simulink model "Traction_Test"  (R2019b)
settings: configuration reference "ConfigSet_TractionSystem_Reference" (kept outside this file)
PostLoadFcn:
  | set_up_test_model()
undefined symbols (not defined in the file): DiscIntNeverNeededParam, ElectricalSystem, Enabled, MaxVehicles, Orientation, Type, VehicleType, WheelDiameter, Z_TractionSystemPrm
libraries: TestBenchLib x27, simulink x2, VectorOperationsLib x1, MathOperationsLib x1
settings Model: EnablePacing=on  PacingRate=0.100000  OrderedModelArguments=off  Creator=lonkaran  LastModifiedBy=ext-nadpurob
settings ConfigSetRef: SourceName=ConfigSet_TractionSystem_Reference  SourceLocation=Base Workspace

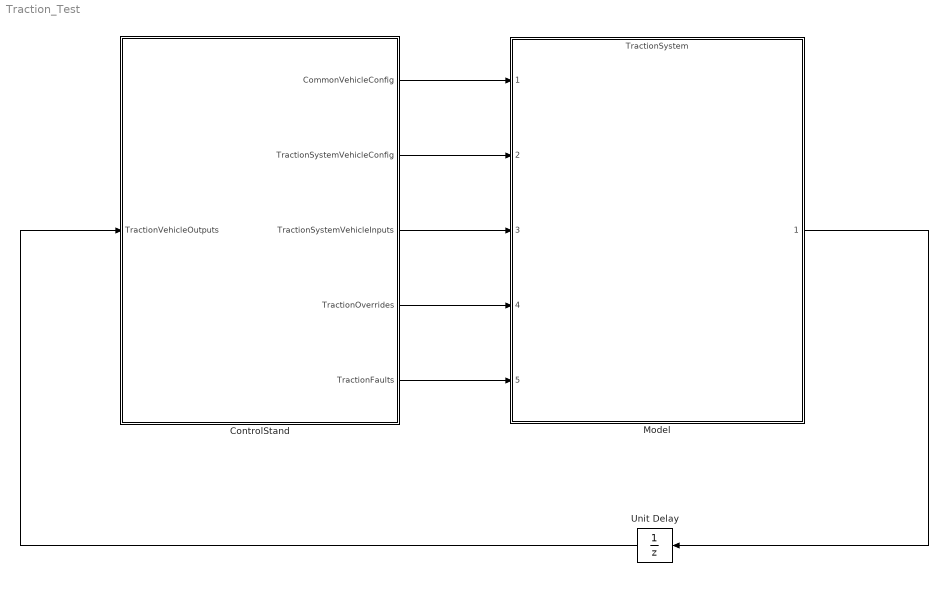
== system Traction_Test ==
  ControlStand : Subsystem
  Model : ModelReference  ModelNameDialog=TractionSystem.slx  ParameterArgumentNames=Prm_TractionSystem  ParameterArgumentValues=[Z_TractionSystemPrm]  UsingDefaultArgumentValue=0  SimulationMode=Normal  ModelReferenceVersion=1.647
  Unit Delay : UnitDelay  SampleTime=-1  HasFrameUpgradeWarning=on
  wires:
  Model/1 -> Unit Delay/1
  Unit Delay/1 -> ControlStand/1(TractionVehicleOutputs)
  ControlStand/1(CommonVehicleConfig) -> Model/1
  ControlStand/2(TractionSystemVehicleConfig) -> Model/2
  ControlStand/3(TractionSystemVehicleInputs) -> Model/3
  ControlStand/4(TractionOverrides) -> Model/4
  ControlStand/5(TractionFaults) -> Model/5

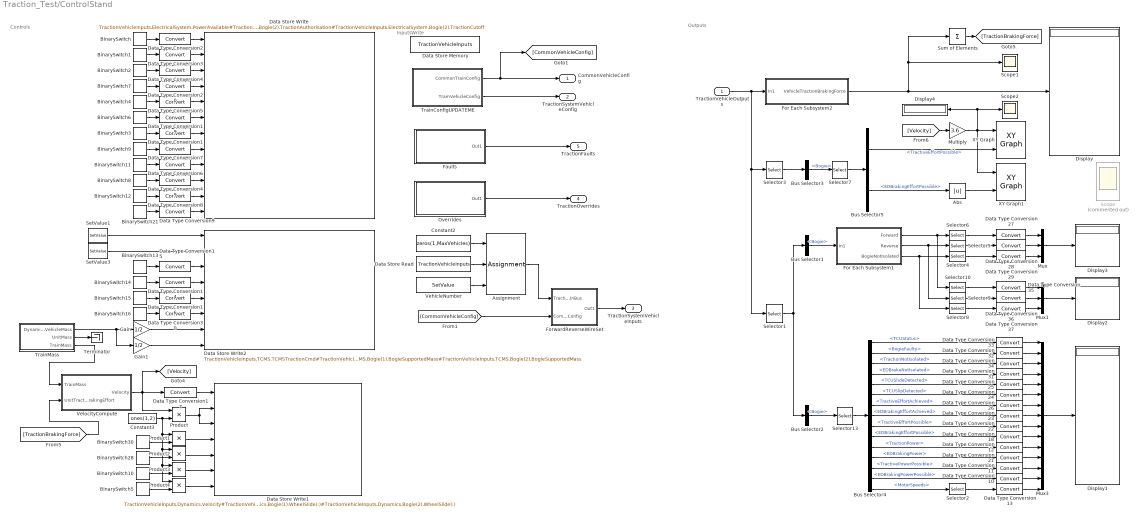
== system Traction_Test/ControlStand ==
  note: Outputs
  note: InputsWrite
  note: Controls
  TractionVehicleOutputs : Inport
  Abs : Abs
  Assignment : Assignment  DiagnosticForDimensions=Warning  IndexOptions=Index vector (port)  Indices=1  OutputSizes=1
  BinarySwitch{,1,3..4,6..9,12} (9 alike) : TestBenchLib/BinarySwitch  value=1  init_value=1  block_colour=[0 1 0]  WorkspaceVarName=0
      settings: SourceProductName=Sydac Utilities
  BinarySwitch{2,5,10..11,13..16,21,28,30} (11 alike) : TestBenchLib/BinarySwitch  value=0  init_value=0  block_colour=[0 1 0]  WorkspaceVarName=0
      settings: SourceProductName=Sydac Utilities
  Bus Selector1 : BusSelector  OutputSignals=TractionControl.ElectricalSystem.Bogie
  Bus Selector2 : BusSelector  OutputSignals=TractionControl.TCMS.Bogie
  Bus Selector3 : BusSelector  OutputSignals=TractionControl.TCMS.Bogie
  Bus Selector4 : BusSelector  OutputSignals=TCUStatus,BogieFaulty,TractionNotIsolated,EDBrakeNotIsolated,TCUSlideDetected,TCUSlipDetected,TractiveEffortAchieved,EDBrakingEffortAchieved,TractiveEffortPossible,EDBrakingEffortPossible,TractionPower,EDBrakingPower,TractivePowerPossible,EDBrakingPowerPossible,MotorSpeeds
  Bus Selector5 : BusSelector  OutputSignals=TractiveEffortPossible,EDBrakingEffortPossible
  Constant2 : Constant  Value=zeros(1,MaxVehicles)  OutDataTypeStr=Bus: BD_TractionSystem_In_Vehicle
  Constant3 : Constant  Value=ones(1,2)
  Data Store Memory : DataStoreMemory  DataStoreName=TractionVehicleInputs  ReadBeforeWriteMsg=warning  WriteAfterWriteMsg=warning  WriteAfterReadMsg=warning  ShowAdditionalParam=off  OutDataTypeStr=Bus: BD_TractionSystem_In_Vehicle
  Data Store Read : DataStoreRead  DataStoreName=TractionVehicleInputs  DataStoreElements=TractionVehicleInputs
  Data Store Write : DataStoreWrite  DataStoreName=TractionVehicleInputs  DataStoreElements=TractionVehicleInputs.ElectricalSystem.PowerAvailable#TractionVehicleInputs.ElectricalSystem.ForwardTW#TractionVehicleInputs.ElectricalSystem.ReverseTW#TractionVehicleInputs.ElectricalSystem.TractionActiveTW#TractionVehicleInputs.ElectricalSystem.NoEmergencyBrakeActiveTW#TractionVehicleInputs.ElectricalSystem.VCBState#TractionVehicleInputs.ElectricalSystem.Bogie(1).TCUPower#TractionVehicleInputs.ElectricalSystem.Bogie(1).TractionAuthorisation#TractionVehicleInputs.ElectricalSystem.Bogie(1).TractionCutoff#TractionVehicleInputs.ElectricalSystem.Bogie(2).TCUPower#TractionVehicleInputs.ElectricalSystem.Bogie(2).TractionAuthorisation#TractionVehicleInputs.ElectricalSystem.Bogie(2).TractionCutoff
  Data Store Write1 : DataStoreWrite  DataStoreName=TractionVehicleInputs  DataStoreElements=TractionVehicleInputs.Dynamics.Velocity#TractionVehicleInputs.Dynamics.Bogie(1).WheelSpeed(:)#TractionVehicleInputs.Dynamics.Bogie(2).WheelSpeed(:)#TractionVehicleInputs.Dynamics.Bogie(1).WheelSlip(:)#TractionVehicleInputs.Dynamics.Bogie(2).WheelSlip(:)#TractionVehicleInputs.Dynamics.Bogie(1).WheelSlide(:)#TractionVehicleInputs.Dynamics.Bogie(2).WheelSlide(:)
  Data Store Write2 : DataStoreWrite  DataStoreName=TractionVehicleInputs  DataStoreElements=TractionVehicleInputs.TCMS.TCMSTractionCmd#TractionVehicleInputs.TCMS.TCMSEDBrakingCmd#TractionVehicleInputs.TCMS.Bogie(1).TCMSTractionInhibit#TractionVehicleInputs.TCMS.Bogie(2).TCMSTractionInhibit#TractionVehicleInputs.TCMS.Bogie(1).TCMSDynamicBrakingInhibit#TractionVehicleInputs.TCMS.Bogie(2).TCMSDynamicBrakingInhibit#TractionVehicleInputs.TCMS.Bogie(1).BogieSupportedMass#TractionVehicleInputs.TCMS.Bogie(2).BogieSupportedMass
  Data Type Conversion{1..37,49} (38 alike) : DataTypeConversion
  Display{,1..4} (5 alike) : Display
  Faults : Subsystem
  For Each Subsystem1 : Subsystem  TreatAsAtomicUnit=on
  For Each Subsystem2 : Subsystem  TreatAsAtomicUnit=on
  ForwardReverseWireSet : Subsystem
  Gain : Gain  Gain=1/2
  Gain1 : Gain  Gain=1/2
  Multiply : Gain  Gain=3.6
  Mux : Mux  Inputs=3
  Mux1 : Mux  Inputs=3
  Mux3 : Mux  Inputs=15
  Overrides : Subsystem
  Product{,1..4} (5 alike) : Product
  Scope : Scope  Commented=on  NumInputPorts=2
  Scope1 : Scope
  Scope2 : Scope
  Selector1 : Selector  InputPortWidth=MaxVehicles  IndexOptions=Index vector (dialog)  Indices=[1]  OutputSizes=1
  Selector10 : Selector  InputPortWidth=2  IndexOptions=Index vector (dialog)  Indices=2  OutputSizes=1
  Selector{2,4..7,13} (6 alike) : Selector  InputPortWidth=2  IndexOptions=Index vector (dialog)  Indices=[1]  OutputSizes=1
  Selector3 : Selector  InputPortWidth=MaxVehicles  IndexOptions=Index vector (dialog)  Indices=[1]  OutputSizes=1
  Selector8 : Selector  InputPortWidth=2  IndexOptions=Index vector (dialog)  Indices=2  OutputSizes=1
  Selector9 : Selector  InputPortWidth=2  IndexOptions=Index vector (dialog)  Indices=2  OutputSizes=1
  SetValue1 : TestBenchLib/SetValue  value=0  init_value=0  WorkspaceVarName=0
      settings: SourceProductName=Sydac Utilities
  SetValue3 : TestBenchLib/SetValue  value=0  init_value=0  WorkspaceVarName=0
      settings: SourceProductName=Sydac Utilities
  Sum of Elements : Sum  Inputs=+
  Terminator : Terminator
  TrainConfigUPDATEME : Subsystem
  TrainMass : Subsystem  mask(Set Train Mass){AW=2}
      mask prompts: AW "Number of units (1 or 2)"
      mask help:
      | In kg, the vehicles' tare masses are:
      |
      | Z1	60 000
      | Z2	52 000
      | Z3	46 000
      | Z4	45 550
      | Single Unit	361 550
      | Multi Unit	723 100
  VehicleNumber : TestBenchLib/SetValue  value=[1:MaxVehicles]  init_value=[1:MaxVehicles]  WorkspaceVarName=0
      settings: SourceProductName=Sydac Utilities
  VelocityCompute : Subsystem  mask{InitSpeed=0}
      mask prompts: InitSpeed "Initial Forward Speed [km/h]"
  XY Graph : simulink/Sinks/XY Graph  xmin=0  xmax=140  ymin=0  ymax=1e5  st=-1
  XY Graph1 : simulink/Sinks/XY Graph  xmin=0  xmax=140  ymin=0  ymax=1e5  st=-1
  CommonVehicleConfig : Outport
  TractionSystemVehicleConfig : Outport  Port=2
  TractionSystemVehicleInputs : Outport  Port=3
  TractionOverrides : Outport  Port=4
  TractionFaults : Outport  Port=5
  wires:
  Faults/1(Out1) -> TractionFaults/1
  Overrides/1(Out1) -> TractionOverrides/1
  TrainConfigUPDATEME/1(CommonTrainConfig) -> [CommonVehicleConfig], CommonVehicleConfig/1
  TrainConfigUPDATEME/2(TramVehicleConfig) -> TractionSystemVehicleConfig/1
  VehicleNumber/1 -> Assignment/3
  Constant2/1 -> Assignment/1
  Data Store Read/1 -> Assignment/2
  BinarySwitch/1 -> Data Type Conversion2/1
  BinarySwitch1/1 -> Data Type Conversion3/1
  BinarySwitch2/1 -> Data Type Conversion4/1
  BinarySwitch11/1 -> Data Type Conversion6/1
  BinarySwitch12/1 -> Data Type Conversion8/1
  BinarySwitch21/1 -> Data Type Conversion9/1
  BinarySwitch3/1 -> Data Type Conversion1/1
  BinarySwitch9/1 -> Data Type Conversion7/1
  Constant3/1 -> Product4/1, Product3/1, Product2/1, Product1/1, Product/2
  Product/1 -> Data Store Write1/2, Data Store Write1/3
  Data Type Conversion1/1 -> Data Store Write/7
  Data Type Conversion2/1 -> Data Store Write/1
  Data Type Conversion3/1 -> Data Store Write/2
  Data Type Conversion4/1 -> Data Store Write/3
  Data Type Conversion5/1 -> Data Store Write/5
  Data Type Conversion6/1 -> Data Store Write/9
  Data Type Conversion8/1 -> Data Store Write/11
  Data Type Conversion9/1 -> Data Store Write/12
  For Each Subsystem2/1(VehicleTractionBrakingForce) -> Scope1/1, Sum of Elements/1, Display/1
  Multiply/1 -> XY Graph1/1, XY Graph/1, Scope2/1, Display4/1
  Data Type Conversion17/1 -> Data Store Write1/1
  BinarySwitch4/1 -> Data Type Conversion5/1
  Data Type Conversion20/1 -> Data Store Write/4
  Data Type Conversion19/1 -> Data Store Write/6
  BinarySwitch6/1 -> Data Type Conversion19/1
  BinarySwitch7/1 -> Data Type Conversion20/1
  [Velocity] -> Multiply/1
  TractionVehicleOutputs/1 -> Selector3/1, Selector1/1, For Each Subsystem2/1(In1)
  Selector1/1 -> Bus Selector2/1, Bus Selector1/1
  Bus Selector1/1 -> For Each Subsystem1/1(In1)  "<Bogie>"
  Mux3/1 -> Display1/1
  Mux/1 -> Display3/1
  Data Type Conversion27/1 -> Mux/1
  Data Type Conversion28/1 -> Mux/2
  VelocityCompute/1(Velocity) -> Data Type Conversion17/1, Product/1, [Velocity]
  [TractionBrakingForce] -> VelocityCompute/2(UnitTractionBrakingEffort)
  TrainMass/3(TrainMass) -> VelocityCompute/1(TrainMass)
  Assignment/1 -> ForwardReverseWireSet/1(TractionInBus)
  [CommonVehicleConfig] -> ForwardReverseWireSet/2(CommonConfig)
  ForwardReverseWireSet/1(Out1) -> TractionSystemVehicleInputs/1
  BinarySwitch8/1 -> Data Type Conversion49/1
  Data Type Conversion49/1 -> Data Store Write/10
  Data Type Conversion7/1 -> Data Store Write/8
  SetValue1/1 -> Data Store Write2/1
  SetValue3/1 -> Data Store Write2/2
  For Each Subsystem1/2(Reverse) -> Selector9/1, Selector5/1
  For Each Subsystem1/3(BogieNotIsolated) -> Selector8/1, Selector4/1
  Data Type Conversion29/1 -> Mux/3
  Selector4/1 -> Data Type Conversion29/1
  Selector5/1 -> Data Type Conversion28/1
  Selector6/1 -> Data Type Conversion27/1
  Selector10/1 -> Data Type Conversion35/1
  Selector9/1 -> Data Type Conversion36/1
  Selector8/1 -> Data Type Conversion37/1
  Data Type Conversion37/1 -> Mux1/3
  Data Type Conversion36/1 -> Mux1/2
  Data Type Conversion35/1 -> Mux1/1
  Mux1/1 -> Display2/1
  For Each Subsystem1/1(Forward) -> Selector10/1, Selector6/1
  TrainMass/1(DynamicsVehicleMass) -> Gain1/1, Gain/1
  Sum of Elements/1 -> [TractionBrakingForce]
  BinarySwitch30/1 -> Product1/2
  BinarySwitch28/1 -> Product2/2
  BinarySwitch10/1 -> Product3/2
  BinarySwitch5/1 -> Product4/2
  Product1/1 -> Data Store Write1/4
  Product2/1 -> Data Store Write1/5
  Product3/1 -> Data Store Write1/6
  Product4/1 -> Data Store Write1/7
  TrainMass/2(UnitMass) -> Terminator/1
  Gain/1 -> Data Store Write2/7
  Gain1/1 -> Data Store Write2/8
  BinarySwitch13/1 -> Data Type Conversion15/1
  BinarySwitch14/1 -> Data Type Conversion14/1
  BinarySwitch16/1 -> Data Type Conversion30/1
  BinarySwitch15/1 -> Data Type Conversion16/1
  Bus Selector2/1 -> Selector13/1  "<Bogie>"
  Selector13/1 -> Bus Selector4/1
  Bus Selector5/1 -> XY Graph/2  "<TractiveEffortPossible>"
  Abs/1 -> XY Graph1/2
  Bus Selector4/15 -> Selector2/1  "<MotorSpeeds>"
  Selector2/1 -> Data Type Conversion13/1
  Data Type Conversion13/1 -> Mux3/15
  Bus Selector3/1 -> Selector7/1  "<Bogie>"
  Selector3/1 -> Bus Selector3/1
  Bus Selector5/2 -> Abs/1  "<EDBrakingEffortPossible>"
  Selector7/1 -> Bus Selector5/1
  Data Type Conversion15/1 -> Data Store Write2/3
  Data Type Conversion16/1 -> Data Store Write2/5
  Data Type Conversion30/1 -> Data Store Write2/6
  Data Type Conversion14/1 -> Data Store Write2/4
  Data Type Conversion21/1 -> Mux3/12
  Data Type Conversion10/1 -> Mux3/14
  Data Type Conversion11/1 -> Mux3/13
  Data Type Conversion12/1 -> Mux3/11
  Data Type Conversion18/1 -> Mux3/10
  Bus Selector4/10 -> Data Type Conversion18/1  "<EDBrakingEffortPossible>"
  Bus Selector4/11 -> Data Type Conversion12/1  "<TractionPower>"
  Bus Selector4/12 -> Data Type Conversion21/1  "<EDBrakingPower>"
  Bus Selector4/13 -> Data Type Conversion11/1  "<TractivePowerPossible>"
  Bus Selector4/14 -> Data Type Conversion10/1  "<EDBrakingPowerPossible>"
  Bus Selector4/9 -> Data Type Conversion22/1  "<TractiveEffortPossible>"
  Bus Selector4/8 -> Data Type Conversion23/1  "<EDBrakingEffortAchieved>"
  Bus Selector4/7 -> Data Type Conversion26/1  "<TractiveEffortAchieved>"
  Bus Selector4/6 -> Data Type Conversion24/1  "<TCUSlipDetected>"
  Bus Selector4/5 -> Data Type Conversion25/1  "<TCUSlideDetected>"
  Data Type Conversion25/1 -> Mux3/5
  Data Type Conversion24/1 -> Mux3/6
  Data Type Conversion23/1 -> Mux3/8
  Data Type Conversion22/1 -> Mux3/9
  Data Type Conversion26/1 -> Mux3/7
  Data Type Conversion34/1 -> Mux3/3
  Data Type Conversion31/1 -> Mux3/4
  Data Type Conversion32/1 -> Mux3/2
  Data Type Conversion33/1 -> Mux3/1
  Bus Selector4/1 -> Data Type Conversion33/1  "<TCUStatus>"
  Bus Selector4/2 -> Data Type Conversion32/1  "<BogieFaulty>"
  Bus Selector4/3 -> Data Type Conversion34/1  "<TractionNotIsolated>"
  Bus Selector4/4 -> Data Type Conversion31/1  "<EDBrakeNotIsolated>"

== system Traction_Test/ControlStand/Faults ==
  Constant1 : Constant  Value=zeros(1,MaxVehicles)  OutDataTypeStr=Bus: BD_TractionSystem_In_Faults
  Out1 : Outport  VectorParamsAs1DForOutWhenUnconnected=off
  wires:
  Constant1/1 -> Out1/1

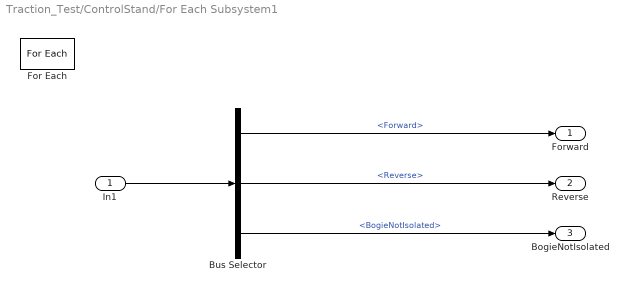
== system Traction_Test/ControlStand/For Each Subsystem1 ==
  In1 : Inport  Partition=on  PartitionDimension=1  PartitionWidth=1  PartitionOffset=0
  Bus Selector : BusSelector  OutputSignals=Forward,Reverse,BogieNotIsolated
  For Each : ForEach  DisableCoverage=on
  Forward : Outport  ConcatenationDimension=1
  Reverse : Outport  Port=2  ConcatenationDimension=1
  BogieNotIsolated : Outport  Port=3  ConcatenationDimension=1
  wires:
  Bus Selector/1 -> Forward/1  "<Forward>"
  In1/1 -> Bus Selector/1
  Bus Selector/2 -> Reverse/1  "<Reverse>"
  Bus Selector/3 -> BogieNotIsolated/1  "<BogieNotIsolated>"

== system Traction_Test/ControlStand/For Each Subsystem2 ==
  In1 : Inport  Partition=on  PartitionDimension=1  PartitionWidth=1  PartitionOffset=0
  Bus Selector : BusSelector  OutputSignals=Dynamics.TractionBrakingForce
  For Each : ForEach  DisableCoverage=on
  Sum of Elements : Sum  Inputs=+
  VehicleTractionBrakingForce : Outport  ConcatenationDimension=1
  wires:
  In1/1 -> Bus Selector/1
  Bus Selector/1 -> Sum of Elements/1  "<TractionBrakingForce>"
  Sum of Elements/1 -> VehicleTractionBrakingForce/1

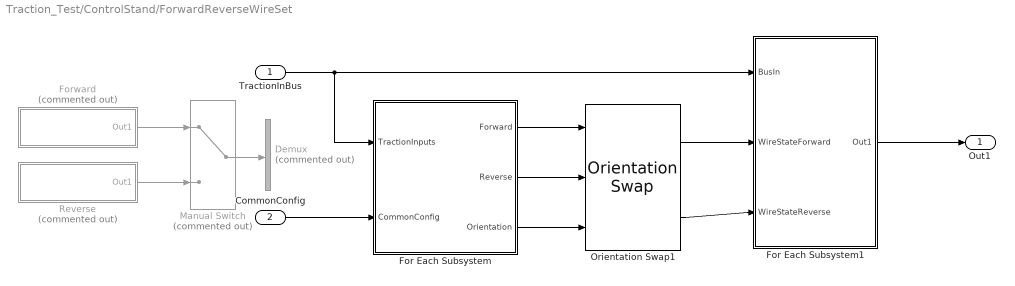
== system Traction_Test/ControlStand/ForwardReverseWireSet ==
  TractionInBus : Inport
  CommonConfig : Inport  Port=2
  Demux : Demux  Commented=on  Outputs=2
  For Each Subsystem : Subsystem  TreatAsAtomicUnit=on
  For Each Subsystem1 : Subsystem  TreatAsAtomicUnit=on
  Forward : Subsystem  Commented=on
  Manual Switch : ManualSwitch  Commented=on
  Orientation Swap1 : VectorOperationsLib/Orientation Swap
      settings: SourceProductName=Sydac Utilities
  Reverse : Subsystem  Commented=on
  Out1 : Outport
  wires:
  Reverse/1(Out1) -> Manual Switch/2
  For Each Subsystem/3(Orientation) -> Orientation Swap1/3
  For Each Subsystem/2(Reverse) -> Orientation Swap1/2
  For Each Subsystem/1(Forward) -> Orientation Swap1/1
  Manual Switch/1 -> Demux/1
  For Each Subsystem1/1(Out1) -> Out1/1
  Forward/1(Out1) -> Manual Switch/1
  Orientation Swap1/2 -> For Each Subsystem1/3(WireStateReverse)
  Orientation Swap1/1 -> For Each Subsystem1/2(WireStateForward)
  TractionInBus/1 -> For Each Subsystem1/1(BusIn), For Each Subsystem/1(TractionInputs)
  CommonConfig/1 -> For Each Subsystem/2(CommonConfig)

== system Traction_Test/ControlStand/Overrides ==
  Constant1 : Constant  Value=zeros(1,MaxVehicles)  OutDataTypeStr=Bus: BD_TractionSystem_In_Overrides
  Out1 : Outport
  wires:
  Constant1/1 -> Out1/1

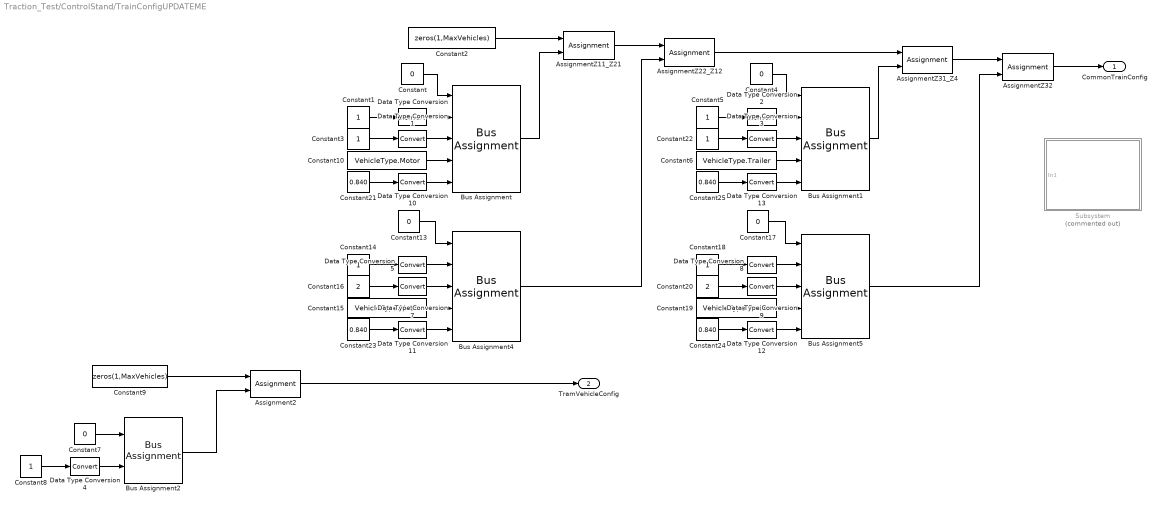
== system Traction_Test/ControlStand/TrainConfigUPDATEME ==
  Assignment2 : Assignment  DiagnosticForDimensions=Warning  IndexOptions=Index vector (dialog)  Indices=[1,3,5,6,8]  OutputSizes=1
  AssignmentZ11_Z21 : Assignment  DiagnosticForDimensions=Warning  IndexOptions=Index vector (dialog)  Indices=[1,3,5]  OutputSizes=1
  AssignmentZ22_Z12 : Assignment  DiagnosticForDimensions=Warning  IndexOptions=Index vector (dialog)  Indices=[6,8]  OutputSizes=1
  AssignmentZ31_Z4 : Assignment  DiagnosticForDimensions=Warning  IndexOptions=Index vector (dialog)  Indices=[2,4]  OutputSizes=1
  AssignmentZ32 : Assignment  DiagnosticForDimensions=Warning  IndexOptions=Index vector (dialog)  Indices=[7]  OutputSizes=1
  Bus Assignment{,1,4..5} (4 alike) : BusAssignment  AssignedSignals=Enabled,Orientation,Type,WheelDiameter
  Bus Assignment2 : BusAssignment  AssignedSignals=HasMotors
  Constant{,4,13,17} (4 alike) : Constant  Value=0  OutDataTypeStr=Bus: BD_CommonTrain_Cfg_Vehicle
  Constant{1,3,5,8,14,18,22} (7 alike) : Constant
  Constant10 : Constant  Value=VehicleType.Motor
  Constant15 : Constant  Value=VehicleType.Motor
  Constant16 : Constant  Value=2
  Constant19 : Constant  Value=VehicleType.Trailer
  Constant2 : Constant  Value=zeros(1,MaxVehicles)  OutDataTypeStr=Bus: BD_CommonTrain_Cfg_Vehicle
  Constant20 : Constant  Value=2
  Constant{21,23..25} (4 alike) : Constant  Value=0.840
  Constant6 : Constant  Value=VehicleType.Trailer
  Constant7 : Constant  Value=0  OutDataTypeStr=Bus: BD_TractionSystem_Cfg_Vehicle
  Constant9 : Constant  Value=zeros(1,MaxVehicles)  OutDataTypeStr=Bus: BD_TractionSystem_Cfg_Vehicle
  Data Type Conversion{,1..5,7..13} (13 alike) : DataTypeConversion
  Subsystem : Subsystem  Commented=on
  CommonTrainConfig : Outport  VectorParamsAs1DForOutWhenUnconnected=off
  TramVehicleConfig : Outport  Port=2  VectorParamsAs1DForOutWhenUnconnected=off
  wires:
  Constant/1 -> Bus Assignment/1
  Constant1/1 -> Data Type Conversion/1
  Constant2/1 -> AssignmentZ11_Z21/1
  Bus Assignment/1 -> AssignmentZ11_Z21/2
  Data Type Conversion/1 -> Bus Assignment/2
  AssignmentZ32/1 -> CommonTrainConfig/1
  Constant3/1 -> Data Type Conversion1/1
  Data Type Conversion1/1 -> Bus Assignment/3
  Data Type Conversion4/1 -> Bus Assignment2/2
  Bus Assignment2/1 -> Assignment2/2
  Constant9/1 -> Assignment2/1
  Constant8/1 -> Data Type Conversion4/1
  Constant7/1 -> Bus Assignment2/1
  Constant10/1 -> Bus Assignment/4
  Constant15/1 -> Bus Assignment4/4
  Data Type Conversion7/1 -> Bus Assignment4/3
  Constant16/1 -> Data Type Conversion7/1
  Data Type Conversion5/1 -> Bus Assignment4/2
  Bus Assignment4/1 -> AssignmentZ22_Z12/2
  AssignmentZ11_Z21/1 -> AssignmentZ22_Z12/1
  Constant14/1 -> Data Type Conversion5/1
  Constant13/1 -> Bus Assignment4/1
  Constant17/1 -> Bus Assignment5/1
  Constant18/1 -> Data Type Conversion8/1
  AssignmentZ31_Z4/1 -> AssignmentZ32/1
  Bus Assignment5/1 -> AssignmentZ32/2
  Data Type Conversion8/1 -> Bus Assignment5/2
  Constant20/1 -> Data Type Conversion9/1
  Data Type Conversion9/1 -> Bus Assignment5/3
  Constant19/1 -> Bus Assignment5/4
  Constant6/1 -> Bus Assignment1/4
  Data Type Conversion3/1 -> Bus Assignment1/3
  Constant22/1 -> Data Type Conversion3/1
  Data Type Conversion2/1 -> Bus Assignment1/2
  Bus Assignment1/1 -> AssignmentZ31_Z4/2
  AssignmentZ22_Z12/1 -> AssignmentZ31_Z4/1
  Constant5/1 -> Data Type Conversion2/1
  Constant4/1 -> Bus Assignment1/1
  Constant21/1 -> Data Type Conversion10/1
  Data Type Conversion10/1 -> Bus Assignment/5
  Data Type Conversion11/1 -> Bus Assignment4/5
  Constant23/1 -> Data Type Conversion11/1
  Constant24/1 -> Data Type Conversion12/1
  Data Type Conversion12/1 -> Bus Assignment5/5
  Data Type Conversion13/1 -> Bus Assignment1/5
  Constant25/1 -> Data Type Conversion13/1
  Assignment2/1 -> TramVehicleConfig/1

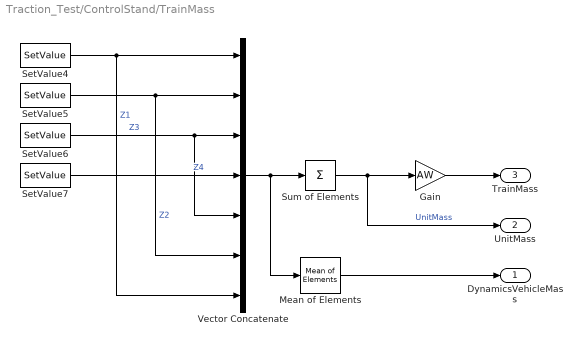
== system Traction_Test/ControlStand/TrainMass ==
  Gain : Gain  Gain=AW
  Mean of Elements : MathOperationsLib/Mean of Elements
      settings: SourceProductName=Math Operations
  SetValue4 : TestBenchLib/SetValue  value=60000  init_value=60000  WorkspaceVarName=0
      settings: SourceProductName=Sydac Utilities
  SetValue5 : TestBenchLib/SetValue  value=52000  init_value=52000  WorkspaceVarName=0
      settings: SourceProductName=Sydac Utilities
  SetValue6 : TestBenchLib/SetValue  value=46000  init_value=46000  WorkspaceVarName=0
      settings: SourceProductName=Sydac Utilities
  SetValue7 : TestBenchLib/SetValue  value=45550  init_value=45550  WorkspaceVarName=0
      settings: SourceProductName=Sydac Utilities
  Sum of Elements : Sum  Inputs=+
  Vector Concatenate : Concatenate  NumInputs=7
  DynamicsVehicleMass : Outport
  UnitMass : Outport  Port=2
  TrainMass : Outport  Port=3
  wires:
  SetValue4/1 -> Vector Concatenate/1, Vector Concatenate/7  "Z1"
  SetValue7/1 -> Vector Concatenate/4  "Z4"
  SetValue5/1 -> Vector Concatenate/2, Vector Concatenate/6  "Z2"
  Gain/1 -> TrainMass/1
  SetValue6/1 -> Vector Concatenate/3, Vector Concatenate/5  "Z3"
  Sum of Elements/1 -> UnitMass/1, Gain/1  "UnitMass"
  Vector Concatenate/1 -> Sum of Elements/1, Mean of Elements/1
  Mean of Elements/1 -> DynamicsVehicleMass/1

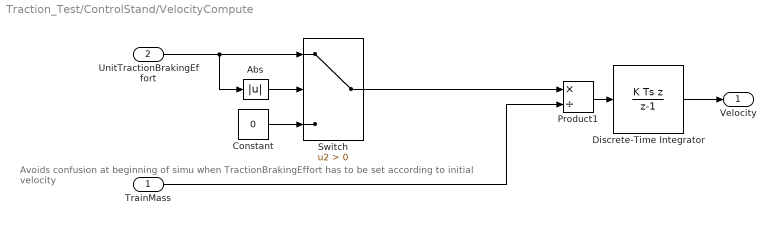
== system Traction_Test/ControlStand/VelocityCompute ==
  note: Avoids confusion at beginning of simu when TractionBrakingEffort has to be set according to initial velocity
  TrainMass : Inport
  UnitTractionBrakingEffort : Inport  Port=2
  Abs : Abs
  Constant : Constant  Value=0
  Discrete-Time Integrator : DiscreteIntegrator  IntegratorMethod=Integration: Backward Euler  InitialCondition=InitSpeed/3.6  SampleTime=-1  LimitOutput=on  UpperSaturationLimit=100  LowerSaturationLimit=-100  ICPrevOutput=DiscIntNeverNeededParam  ICPrevScaledInput=DiscIntNeverNeededParam
  Product1 : Product  Inputs=*/
  Switch : Switch  Criteria=u2 > Threshold
  Velocity : Outport
  wires:
  Constant/1 -> Switch/3
  Abs/1 -> Switch/2
  Discrete-Time Integrator/1 -> Velocity/1
  Product1/1 -> Discrete-Time Integrator/1
  UnitTractionBrakingEffort/1 -> Abs/1, Switch/1
  TrainMass/1 -> Product1/2
  Switch/1 -> Product1/1

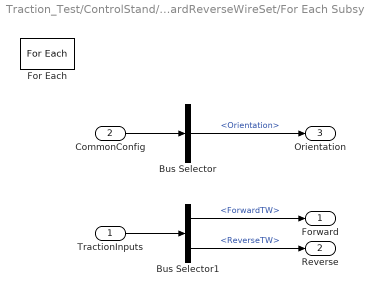
== system Traction_Test/ControlStand/ForwardReverseWireSet/For Each Subsystem ==
  TractionInputs : Inport  Partition=on  PartitionDimension=1  PartitionWidth=1  PartitionOffset=0
  CommonConfig : Inport  Port=2  Partition=on  PartitionDimension=1  PartitionWidth=1  PartitionOffset=0
  Bus Selector : BusSelector  OutputSignals=Orientation
  Bus Selector1 : BusSelector  OutputSignals=ElectricalSystem.ForwardTW,ElectricalSystem.ReverseTW
  For Each : ForEach  DisableCoverage=on
  Forward : Outport  ConcatenationDimension=1
  Reverse : Outport  Port=2  ConcatenationDimension=1
  Orientation : Outport  Port=3  ConcatenationDimension=1
  wires:
  CommonConfig/1 -> Bus Selector/1
  Bus Selector/1 -> Orientation/1  "<Orientation>"
  TractionInputs/1 -> Bus Selector1/1
  Bus Selector1/2 -> Reverse/1  "<ReverseTW>"
  Bus Selector1/1 -> Forward/1  "<ForwardTW>"

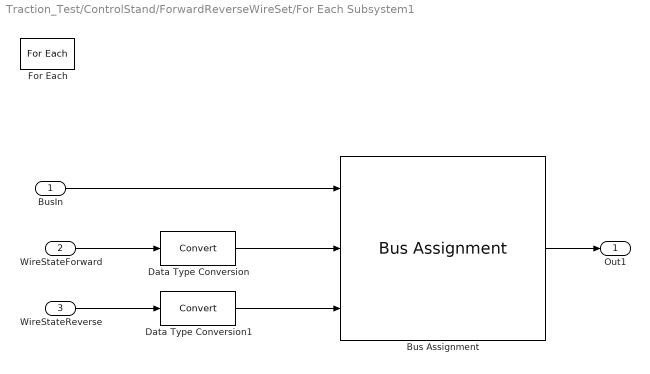
== system Traction_Test/ControlStand/ForwardReverseWireSet/For Each Subsystem1 ==
  BusIn : Inport  Partition=on  PartitionDimension=1  PartitionWidth=1  PartitionOffset=0
  WireStateForward : Inport  Port=2  Partition=on  PartitionDimension=1  PartitionWidth=1  PartitionOffset=0
  WireStateReverse : Inport  Port=3  Partition=on  PartitionDimension=1  PartitionWidth=1  PartitionOffset=0
  Bus Assignment : BusAssignment  AssignedSignals=ElectricalSystem.ForwardTW,ElectricalSystem.ReverseTW
  Data Type Conversion : DataTypeConversion
  Data Type Conversion1 : DataTypeConversion
  For Each : ForEach  DisableCoverage=on
  Out1 : Outport  ConcatenationDimension=1
  wires:
  BusIn/1 -> Bus Assignment/1
  WireStateForward/1 -> Data Type Conversion/1
  WireStateReverse/1 -> Data Type Conversion1/1
  Bus Assignment/1 -> Out1/1
  Data Type Conversion/1 -> Bus Assignment/2
  Data Type Conversion1/1 -> Bus Assignment/3

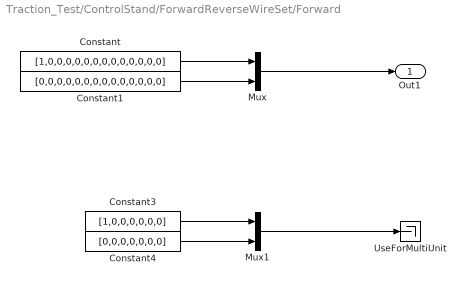
== system Traction_Test/ControlStand/ForwardReverseWireSet/Forward ==
  Constant : Constant  Value=[1,0,0,0,0,0,0,0,0,0,0,0,0,0]
  Constant1 : Constant  Value=[0,0,0,0,0,0,0,0,0,0,0,0,0,0]
  Constant3 : Constant  Value=[1,0,0,0,0,0,0]
  Constant4 : Constant  Value=[0,0,0,0,0,0,0]
  Mux : Mux  Inputs=2
  Mux1 : Mux  Inputs=2
  UseForMultiUnit : Terminator
  Out1 : Outport
  wires:
  Constant/1 -> Mux/1
  Constant1/1 -> Mux/2
  Mux1/1 -> UseForMultiUnit/1
  Mux/1 -> Out1/1
  Constant4/1 -> Mux1/2
  Constant3/1 -> Mux1/1

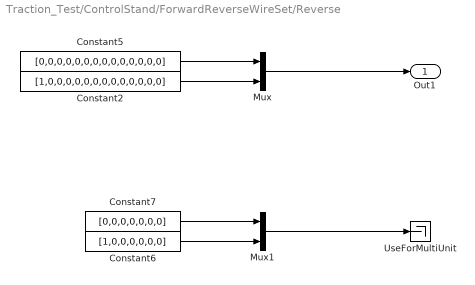
== system Traction_Test/ControlStand/ForwardReverseWireSet/Reverse ==
  Constant2 : Constant  Value=[1,0,0,0,0,0,0,0,0,0,0,0,0,0]
  Constant5 : Constant  Value=[0,0,0,0,0,0,0,0,0,0,0,0,0,0]
  Constant6 : Constant  Value=[1,0,0,0,0,0,0]
  Constant7 : Constant  Value=[0,0,0,0,0,0,0]
  Mux : Mux  Inputs=2
  Mux1 : Mux  Inputs=2
  UseForMultiUnit : Terminator
  Out1 : Outport
  wires:
  Constant7/1 -> Mux1/1
  Constant6/1 -> Mux1/2
  Mux/1 -> Out1/1
  Constant2/1 -> Mux/2
  Constant5/1 -> Mux/1
  Mux1/1 -> UseForMultiUnit/1

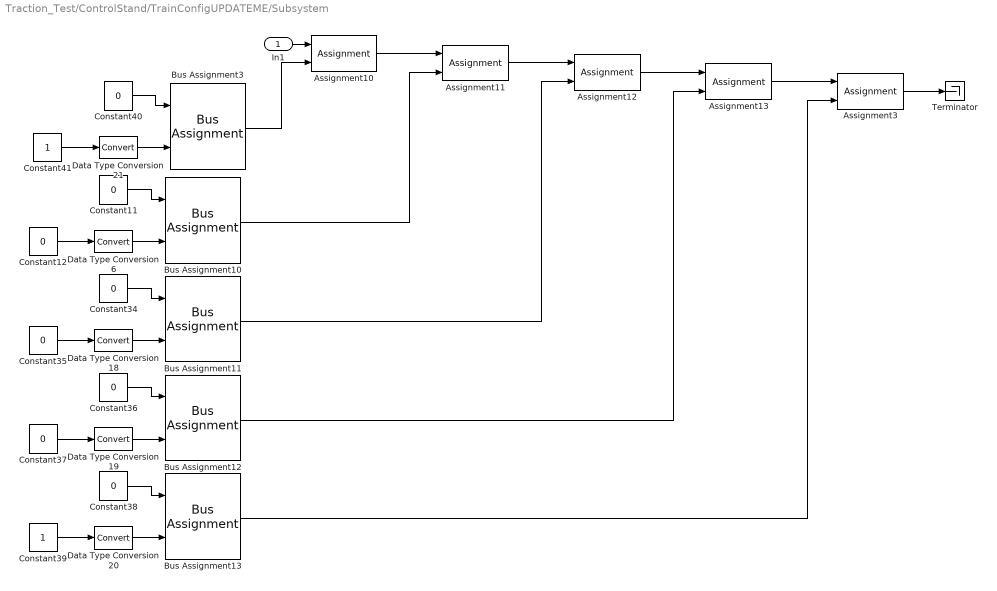
== system Traction_Test/ControlStand/TrainConfigUPDATEME/Subsystem ==
  In1 : Inport
  Assignment10 : Assignment  DiagnosticForDimensions=Warning  IndexOptions=Index vector (dialog)  Indices=6  OutputSizes=1
  Assignment11 : Assignment  DiagnosticForDimensions=Warning  IndexOptions=Index vector (dialog)  Indices=7  OutputSizes=1
  Assignment12 : Assignment  DiagnosticForDimensions=Warning  IndexOptions=Index vector (dialog)  Indices=8  OutputSizes=1
  Assignment13 : Assignment  DiagnosticForDimensions=Warning  IndexOptions=Index vector (dialog)  Indices=9  OutputSizes=1
  Assignment3 : Assignment  DiagnosticForDimensions=Warning  IndexOptions=Index vector (dialog)  Indices=10  OutputSizes=1
  Bus Assignment{3,10..13} (5 alike) : BusAssignment  AssignedSignals=HasMotors
  Constant{11,34,36,38,40} (5 alike) : Constant  Value=0  OutDataTypeStr=Bus: BD_TractionSystem_Cfg_Vehicle
  Constant12 : Constant  Value=0
  Constant35 : Constant  Value=0
  Constant37 : Constant  Value=0
  Constant39 : Constant
  Constant41 : Constant
  Data Type Conversion{6,18..21} (5 alike) : DataTypeConversion
  Terminator : Terminator
  wires:
  Bus Assignment10/1 -> Assignment11/2
  Assignment10/1 -> Assignment11/1
  Constant34/1 -> Bus Assignment11/1
  Assignment12/1 -> Assignment13/1
  Constant39/1 -> Data Type Conversion20/1
  Data Type Conversion18/1 -> Bus Assignment11/2
  Assignment11/1 -> Assignment12/1
  Bus Assignment11/1 -> Assignment12/2
  Constant38/1 -> Bus Assignment13/1
  Bus Assignment13/1 -> Assignment3/2
  Constant37/1 -> Data Type Conversion19/1
  Data Type Conversion19/1 -> Bus Assignment12/2
  Constant36/1 -> Bus Assignment12/1
  Constant41/1 -> Data Type Conversion21/1
  Bus Assignment3/1 -> Assignment10/2
  Constant12/1 -> Data Type Conversion6/1
  Constant11/1 -> Bus Assignment10/1
  Assignment13/1 -> Assignment3/1
  Data Type Conversion20/1 -> Bus Assignment13/2
  Bus Assignment12/1 -> Assignment13/2
  Constant35/1 -> Data Type Conversion18/1
  Data Type Conversion21/1 -> Bus Assignment3/2
  Data Type Conversion6/1 -> Bus Assignment10/2
  Constant40/1 -> Bus Assignment3/1
  Assignment3/1 -> Terminator/1
  In1/1 -> Assignment10/1
